simulink model "LICENTA_2024"  (R2018b)
settings: Solver=FixedStepDiscrete  StartTime=0.0  StopTime=Inf  RelTol=1e-3  EnableMultiTasking=on
values from neighbouring files (symbols this model uses):
  A = -Rs/Ld    (= -2.40983606557)    [licentam18.m]
  const_cuplu = 0.035    [licentam18.m]
  factor_conversie = (1/Rshunt)*(1/10)*(vref/4095)    (= 0.0115122972266)    [licentam18.m]
  FED = uint16(50)    [licentam18.m]
  MaxIter_1_ms_eCAP_wait = MinDetectSpeed_period/T_pos    (= 375)    [licentam18.m]
  pp = 16/2    (= 8)    [licentam18.m]
  RED = uint16(50)    [licentam18.m]
  T_pos = 0.0005    [licentam18.m]
  TBPRD1 = uint16(TPWM/(2*TTBCLK))    [licentam18.m]
  Tf = 0.015    [licentam18.m]
  Tf_spd = 0.01    [licentam18.m]
  Ts = Ts_crt_control    (= 3.33333333333e-05)    [licentam18.m]
  TTBCLK = 1/F    (= 5e-09)    [licentam18.m]
undefined symbols (not defined in the file or in its folder): Down, GPTRIP1SEL, GPTRIP2SEL, K, offset_ADC, radians, TZ1, TZ2, Up
libraries: tiiqmathlib x39, c2802xlib x9, c2837xDlib x6, simulink x5, c280xlib x4, c28xdmclib x2, c2000lib x1
(part 2 of 2)

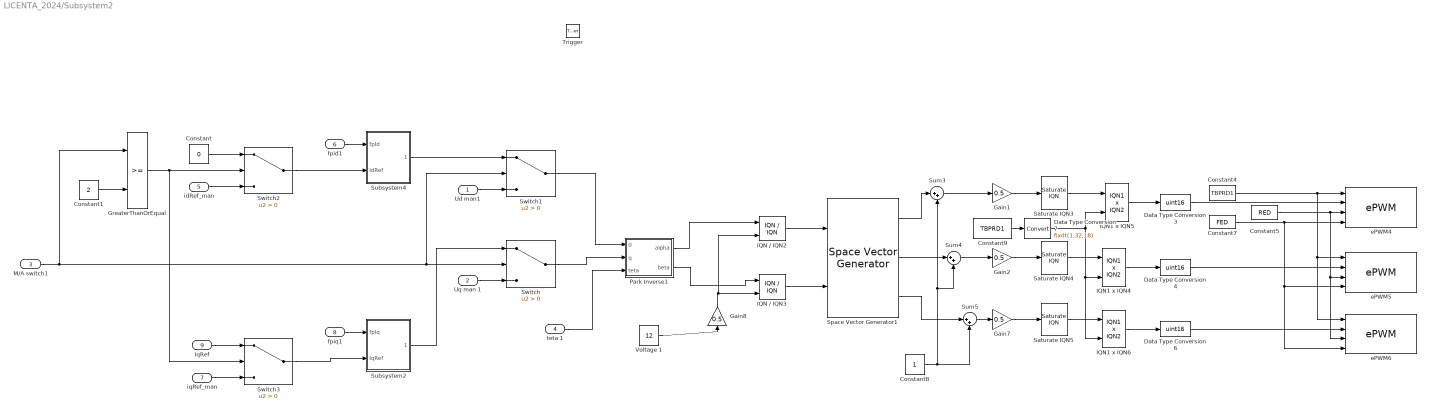
== system LICENTA_2024/Subsystem2 ==
  Ud man1 : Inport
  Uq man 1 : Inport  Port=2
  M/A switch1 : Inport  Port=3
  teta 1 : Inport  Port=4
  idRef_man : Inport  Port=5
  fpid1 : Inport  Port=6
  iqRef_man : Inport  Port=7
  fpiq1 : Inport  Port=8
  IqRef : Inport  Port=9
  Trigger : TriggerPort  TriggerType=function-call  VariantControl=Variant  PortDimensions=1
  Constant : Constant  Value=0
  Constant1 : Constant  Value=2
  Constant4 : Constant  Value=TBPRD1
  Constant5 : Constant  Value=RED
  Constant7 : Constant  Value=FED
  Constant8 : Constant  OutDataTypeStr=fixdt(1,32,24)
  Constant9 : Constant  Value=TBPRD1
  Data Type Conversion3 : DataTypeConversion  OutDataTypeStr=uint16
  Data Type Conversion4 : DataTypeConversion  OutDataTypeStr=uint16
  Data Type Conversion6 : DataTypeConversion  OutDataTypeStr=uint16
  Data Type Conversion7 : DataTypeConversion  OutDataTypeStr=fixdt(1,32,18)
  Gain{1..2,7..8} (4 alike) : Gain  Gain=0.5  OutDataTypeStr=Inherit: Same as input
  GreaterThanOrEqual : RelationalOperator  OutDataTypeStr=boolean  RndMeth=Simplest
  IQN / IQN2 : tiiqmathlib/IQN // IQN
      settings: SourceProductName=Embedded Coder Support Package for Texas Instruments C2000 Processors  SourceProductBaseCode=TIC2000
  IQN / IQN3 : tiiqmathlib/IQN // IQN
      settings: SourceProductName=Embedded Coder Support Package for Texas Instruments C2000 Processors  SourceProductBaseCode=TIC2000
  IQN1 x IQN4 : tiiqmathlib/IQN1 x IQN2  Q=10
      settings: SourceProductName=Embedded Coder Support Package for Texas Instruments C2000 Processors  SourceProductBaseCode=TIC2000
  IQN1 x IQN5 : tiiqmathlib/IQN1 x IQN2  Q=10
      settings: SourceProductName=Embedded Coder Support Package for Texas Instruments C2000 Processors  SourceProductBaseCode=TIC2000
  IQN1 x IQN6 : tiiqmathlib/IQN1 x IQN2  Q=10
      settings: SourceProductName=Embedded Coder Support Package for Texas Instruments C2000 Processors  SourceProductBaseCode=TIC2000
  Park Inverse1 : Subsystem
  Saturate IQN3 : tiiqmathlib/Saturate IQN  pos=0.95  neg=0.05
      settings: SourceProductName=Embedded Coder Support Package for Texas Instruments C2000 Processors  SourceProductBaseCode=TIC2000
  Saturate IQN4 : tiiqmathlib/Saturate IQN  pos=0.95  neg=0.05
      settings: SourceProductName=Embedded Coder Support Package for Texas Instruments C2000 Processors  SourceProductBaseCode=TIC2000
  Saturate IQN5 : tiiqmathlib/Saturate IQN  pos=0.95  neg=0.05
      settings: SourceProductName=Embedded Coder Support Package for Texas Instruments C2000 Processors  SourceProductBaseCode=TIC2000
  Space Vector Generator1 : c28xdmclib/Space Vector Generator
      settings: SourceProductName=Embedded Coder Support Package for Texas Instruments C2000 Processors  SourceProductBaseCode=TIC2000
  Subsystem2 : Subsystem
  Subsystem4 : Subsystem
  Sum3 : Sum  Inputs=|++
  Sum4 : Sum  Inputs=|++
  Sum5 : Sum  Inputs=|++
  Switch{,1..3} (4 alike) : Switch  Criteria=u2 > Threshold
  Voltage 1 : Constant  Value=12  OutDataTypeStr=fixdt(1,32,20)
  ePWM4 : c2802xlib/ePWM  useModule=ePWM1  ePWMxLINKTBPRD=Not Linked  periodUnits=Clock cycles  timerSource=Input port  timerPeriod_clk=TBPRD1+1  timerPeriod_sec=0.0001  tbshadow=Counter equals to zero  countingMode=Up-Down  phaseActiveEnable=Disable  phaseDirection=Count up after sync  phaseActive=0  synchronizationEnable=off  dcaevt1Sync=off  dcbevt1Sync=off  synchronizationOption=Counter equals to zero (CTR=Zero)  clockPrescale=1  HSclockPrescale=1  enswap=off  ePWMxAStatus=on  ePWMxAactionLogic1=Do nothing  ePWMxAactionLogic2=Do nothing  ePWMxAactionLogic3=Clear  ePWMxAactionLogic4=Set  ePWMxAactionLogic5=Do nothing  ePWMxAactionLogic6=Do nothing  ePWMxALoadMode=Load on counter equals to zero (CTR=Zero)  ePWMxACSFenable=off  ePWMxACSFvalue=Forcing disable  ePWMxASFreload=Zero  ePWMxBStatus=off  ePWMxBactionLogic1=Set  ePWMxBactionLogic2=Clear  ePWMxBactionLogic3=Do nothing  ePWMxBactionLogic4=Do nothing  ePWMxBactionLogic5=Clear  ePWMxBactionLogic6=Set  ePWMxBLoadMode=Load on counter equals to zero (CTR=Zero)  ePWMxBCSFenable=off  ePWMxBCSFvalue=Forcing disable  ePWMxBSFreload=Zero  ePWNxBOutWay=off  ePWMxLINKCMPA=Not Linked  CMPAUnits=Clock cycles  CMPASource=Input port  CMPAValue_per=50  CMPAValue_clk=0  enCMPAshadow=Counter equals to zero  ePWMxLINKCMPB=Not Linked  CMPBUnits=Clock cycles  CMPBSource=Specify via dialog  CMPBValue_per=50  CMPBValue_clk=0  enCMPBshadow=Counter equals to zero  ePWMxLINKCMPC=Not Linked  CMPCUnits=Clock cycles  CMPCSource=Specify via dialog  CMPCValue_per=50  CMPCValue_clk=32000  enCMPCshadow=Counter equals to zero  ePWMxLINKCMPD=Not Linked  CMPDUnits=Clock cycles  CMPDSource=Specify via dialog  CMPDValue_per=50  CMPDValue_clk=32000  enCMPDshadow=Counter equals to zero  enableDBePWMxA=on  enableDBePWMxB=on  enhalfcycle=off  DBpolarity=Active high complementary (AHC)  DBedgeDelay=Positive  DBSource_ePWMxA=ePWMxA  DBSource_ePWMxB=ePWMxA  DBperiodSource=Input port  REDperiod=0  FEDperiod=0  adcstartModuleA=on  adcrequestEventA=First event  adcstartEventA=Digital Compare Module A Event 1 start of conversion (DCAEVT1.soc)  adcstartEventA_type2=Counter equals to period (CTR=PRD)  adcstartModuleB=off  adcrequestEventB=First event  adcstartEventB=Counter equals to zero (CTR=Zero)  adcstartEventB_type2=Counter equals to zero (CTR=Zero)  intEn=off  intPrd=First event  intSel=Counter equals to zero (CTR=Zero)  intSel_type2=Counter equals to zero (CTR=Zero)  hrpe=off  enHRPWM=off  HRPWM_LoadMode=Counter equals to period (CTR=PRD)  HRPWM_CTLMode=Duty or Period control mode  HRPWM_EDGMode=Both edge  hrpeb=off  enHRPWMB=off  HRPWM_LoadModeB=Counter equals to zero (CTR=ZERO)  HRPWM_CTLModeB=Duty or Period control mode  HRPWM_EDGModeB=Both edge  enSFO=on  enautoconv=on  chopperEnable=off  chopperFrequency=1  chopperFirstwidth=1  chopperDuty=12.5%  tripZonesource=Specify via dialog  tzselOSHT1=off  tzselOSHT2=off  tzselOSHT3=off  tzselOSHDCAEV1=off  tzselOSHDCBEV1=off  tzselCBC1=off  tzselCBC2=off  tzselCBC3=off  tzselCBCDCAEV2=off  tzselCBCDCBEV2=off  tzselOSHT4=off  tzselOSHT5=off  tzselOSHT6=off  tzselCBC4=off  tzselCBC5=off  tzselCBC6=off  enTzOstIntr=off  enTzCbcIntr=off  enTzDCAEVT1Intr=off  enTzDCAEVT2Intr=off  enTzDCBEVT1Intr=off  enTzDCBEVT2Intr=off  ePWMxAforced=No action  ePWMxBforced=No action  DCAEVT1forced=No action  DCBEVT1forced=No action  DCAEVT2forced=No action  DCBEVT2forced=No action  dcah=Trip Zone 1 input (TZ1)  dcal=Trip Zone 2 input (TZ2)  dcbh=Trip Zone 1 input (TZ1)  dcbl=Trip Zone 2 input (TZ2)  dcah_type2=GPTRIP1SEL/(TZ1)  dcal_type2=GPTRIP2SEL/(TZ2)  dcbh_type2=GPTRIP1SEL/(TZ1)  dcbl_type2=GPTRIP2SEL/(TZ2)  gendcaevt1=Event disabled  gendcaevt2=Event disabled  gendcbevt1=Event disabled  gendcbevt2=Event disabled  dcaevt1src=DCAEVT1 with sync  dcaevt2src=DCAEVT2 with sync  dcbevt1src=DCBEVT1 with sync  dcbevt2src=DCBEVT2 with sync  pulsesel=Counter equals to zero (CTR=Zero)  blankinv=off  blankoffset=0  blankwidth=0  evsrcsel=Filtered version of DCAEVT1 (DCAEVT1FILT)  encape=off  PwmType=C2000_Type4
      settings: SourceProductName=Embedded Coder Support Package for Texas Instruments C2000 Processors
  ePWM5 : c2802xlib/ePWM  useModule=ePWM2  ePWMxLINKTBPRD=Not Linked  periodUnits=Clock cycles  timerSource=Input port  timerPeriod_clk=TBPRD1+1  timerPeriod_sec=0.0001  tbshadow=Counter equals to zero  countingMode=Up-Down  phaseActiveEnable=Disable  phaseDirection=Count up after sync  phaseActive=0  synchronizationEnable=off  dcaevt1Sync=off  dcbevt1Sync=off  synchronizationOption=Counter equals to zero (CTR=Zero)  clockPrescale=1  HSclockPrescale=1  enswap=off  ePWMxAStatus=on  ePWMxAactionLogic1=Do nothing  ePWMxAactionLogic2=Do nothing  ePWMxAactionLogic3=Clear  ePWMxAactionLogic4=Set  ePWMxAactionLogic5=Do nothing  ePWMxAactionLogic6=Do nothing  ePWMxALoadMode=Load on counter equals to zero (CTR=Zero)  ePWMxACSFenable=off  ePWMxACSFvalue=Forcing disable  ePWMxASFreload=Zero  ePWMxBStatus=off  ePWMxBactionLogic1=Set  ePWMxBactionLogic2=Clear  ePWMxBactionLogic3=Do nothing  ePWMxBactionLogic4=Do nothing  ePWMxBactionLogic5=Clear  ePWMxBactionLogic6=Set  ePWMxBLoadMode=Load on counter equals to zero (CTR=Zero)  ePWMxBCSFenable=off  ePWMxBCSFvalue=Forcing disable  ePWMxBSFreload=Zero  ePWNxBOutWay=off  ePWMxLINKCMPA=Not Linked  CMPAUnits=Clock cycles  CMPASource=Input port  CMPAValue_per=50  CMPAValue_clk=0  enCMPAshadow=Counter equals to zero  ePWMxLINKCMPB=Not Linked  CMPBUnits=Clock cycles  CMPBSource=Specify via dialog  CMPBValue_per=50  CMPBValue_clk=0  enCMPBshadow=Counter equals to zero  ePWMxLINKCMPC=Not Linked  CMPCUnits=Clock cycles  CMPCSource=Specify via dialog  CMPCValue_per=50  CMPCValue_clk=32000  enCMPCshadow=Counter equals to zero  ePWMxLINKCMPD=Not Linked  CMPDUnits=Clock cycles  CMPDSource=Specify via dialog  CMPDValue_per=50  CMPDValue_clk=32000  enCMPDshadow=Counter equals to zero  enableDBePWMxA=on  enableDBePWMxB=on  enhalfcycle=off  DBpolarity=Active high complementary (AHC)  DBedgeDelay=Positive  DBSource_ePWMxA=ePWMxA  DBSource_ePWMxB=ePWMxA  DBperiodSource=Input port  REDperiod=0  FEDperiod=0  adcstartModuleA=on  adcrequestEventA=First event  adcstartEventA=Digital Compare Module A Event 1 start of conversion (DCAEVT1.soc)  adcstartEventA_type2=Counter equals to period (CTR=PRD)  adcstartModuleB=off  adcrequestEventB=First event  adcstartEventB=Counter equals to zero (CTR=Zero)  adcstartEventB_type2=Counter equals to zero (CTR=Zero)  intEn=off  intPrd=First event  intSel=Counter equals to zero (CTR=Zero)  intSel_type2=Counter equals to zero (CTR=Zero)  hrpe=off  enHRPWM=off  HRPWM_LoadMode=Counter equals to period (CTR=PRD)  HRPWM_CTLMode=Duty or Period control mode  HRPWM_EDGMode=Both edge  hrpeb=off  enHRPWMB=off  HRPWM_LoadModeB=Counter equals to zero (CTR=ZERO)  HRPWM_CTLModeB=Duty or Period control mode  HRPWM_EDGModeB=Both edge  enSFO=on  enautoconv=on  chopperEnable=off  chopperFrequency=1  chopperFirstwidth=1  chopperDuty=12.5%  tripZonesource=Specify via dialog  tzselOSHT1=off  tzselOSHT2=off  tzselOSHT3=off  tzselOSHDCAEV1=off  tzselOSHDCBEV1=off  tzselCBC1=off  tzselCBC2=off  tzselCBC3=off  tzselCBCDCAEV2=off  tzselCBCDCBEV2=off  tzselOSHT4=off  tzselOSHT5=off  tzselOSHT6=off  tzselCBC4=off  tzselCBC5=off  tzselCBC6=off  enTzOstIntr=off  enTzCbcIntr=off  enTzDCAEVT1Intr=off  enTzDCAEVT2Intr=off  enTzDCBEVT1Intr=off  enTzDCBEVT2Intr=off  ePWMxAforced=No action  ePWMxBforced=No action  DCAEVT1forced=No action  DCBEVT1forced=No action  DCAEVT2forced=No action  DCBEVT2forced=No action  dcah=Trip Zone 1 input (TZ1)  dcal=Trip Zone 2 input (TZ2)  dcbh=Trip Zone 1 input (TZ1)  dcbl=Trip Zone 2 input (TZ2)  dcah_type2=GPTRIP1SEL/(TZ1)  dcal_type2=GPTRIP2SEL/(TZ2)  dcbh_type2=GPTRIP1SEL/(TZ1)  dcbl_type2=GPTRIP2SEL/(TZ2)  gendcaevt1=Event disabled  gendcaevt2=Event disabled  gendcbevt1=Event disabled  gendcbevt2=Event disabled  dcaevt1src=DCAEVT1 with sync  dcaevt2src=DCAEVT2 with sync  dcbevt1src=DCBEVT1 with sync  dcbevt2src=DCBEVT2 with sync  pulsesel=Counter equals to zero (CTR=Zero)  blankinv=off  blankoffset=0  blankwidth=0  evsrcsel=Filtered version of DCAEVT1 (DCAEVT1FILT)  encape=off  PwmType=C2000_Type4
      settings: SourceProductName=Embedded Coder Support Package for Texas Instruments C2000 Processors
  ePWM6 : c2802xlib/ePWM  useModule=ePWM3  ePWMxLINKTBPRD=Not Linked  periodUnits=Clock cycles  timerSource=Input port  timerPeriod_clk=TBPRD1+1  timerPeriod_sec=0.0001  tbshadow=Counter equals to zero  countingMode=Up-Down  phaseActiveEnable=Disable  phaseDirection=Count up after sync  phaseActive=0  synchronizationEnable=off  dcaevt1Sync=off  dcbevt1Sync=off  synchronizationOption=Counter equals to zero (CTR=Zero)  clockPrescale=1  HSclockPrescale=1  enswap=off  ePWMxAStatus=on  ePWMxAactionLogic1=Do nothing  ePWMxAactionLogic2=Do nothing  ePWMxAactionLogic3=Clear  ePWMxAactionLogic4=Set  ePWMxAactionLogic5=Do nothing  ePWMxAactionLogic6=Do nothing  ePWMxALoadMode=Load on counter equals to zero (CTR=Zero)  ePWMxACSFenable=off  ePWMxACSFvalue=Forcing disable  ePWMxASFreload=Zero  ePWMxBStatus=off  ePWMxBactionLogic1=Set  ePWMxBactionLogic2=Clear  ePWMxBactionLogic3=Do nothing  ePWMxBactionLogic4=Do nothing  ePWMxBactionLogic5=Clear  ePWMxBactionLogic6=Set  ePWMxBLoadMode=Load on counter equals to zero (CTR=Zero)  ePWMxBCSFenable=off  ePWMxBCSFvalue=Forcing disable  ePWMxBSFreload=Zero  ePWNxBOutWay=off  ePWMxLINKCMPA=Not Linked  CMPAUnits=Clock cycles  CMPASource=Input port  CMPAValue_per=50  CMPAValue_clk=0  enCMPAshadow=Counter equals to zero  ePWMxLINKCMPB=Not Linked  CMPBUnits=Clock cycles  CMPBSource=Specify via dialog  CMPBValue_per=50  CMPBValue_clk=0  enCMPBshadow=Counter equals to zero  ePWMxLINKCMPC=Not Linked  CMPCUnits=Clock cycles  CMPCSource=Specify via dialog  CMPCValue_per=50  CMPCValue_clk=32000  enCMPCshadow=Counter equals to zero  ePWMxLINKCMPD=Not Linked  CMPDUnits=Clock cycles  CMPDSource=Specify via dialog  CMPDValue_per=50  CMPDValue_clk=32000  enCMPDshadow=Counter equals to zero  enableDBePWMxA=on  enableDBePWMxB=on  enhalfcycle=off  DBpolarity=Active high complementary (AHC)  DBedgeDelay=Positive  DBSource_ePWMxA=ePWMxA  DBSource_ePWMxB=ePWMxA  DBperiodSource=Input port  REDperiod=0  FEDperiod=0  adcstartModuleA=on  adcrequestEventA=First event  adcstartEventA=Digital Compare Module A Event 1 start of conversion (DCAEVT1.soc)  adcstartEventA_type2=Counter equals to period (CTR=PRD)  adcstartModuleB=off  adcrequestEventB=First event  adcstartEventB=Counter equals to zero (CTR=Zero)  adcstartEventB_type2=Counter equals to zero (CTR=Zero)  intEn=off  intPrd=First event  intSel=Counter equals to zero (CTR=Zero)  intSel_type2=Counter equals to zero (CTR=Zero)  hrpe=off  enHRPWM=off  HRPWM_LoadMode=Counter equals to period (CTR=PRD)  HRPWM_CTLMode=Duty or Period control mode  HRPWM_EDGMode=Both edge  hrpeb=off  enHRPWMB=off  HRPWM_LoadModeB=Counter equals to zero (CTR=ZERO)  HRPWM_CTLModeB=Duty or Period control mode  HRPWM_EDGModeB=Both edge  enSFO=on  enautoconv=on  chopperEnable=off  chopperFrequency=1  chopperFirstwidth=1  chopperDuty=12.5%  tripZonesource=Specify via dialog  tzselOSHT1=off  tzselOSHT2=off  tzselOSHT3=off  tzselOSHDCAEV1=off  tzselOSHDCBEV1=off  tzselCBC1=off  tzselCBC2=off  tzselCBC3=off  tzselCBCDCAEV2=off  tzselCBCDCBEV2=off  tzselOSHT4=off  tzselOSHT5=off  tzselOSHT6=off  tzselCBC4=off  tzselCBC5=off  tzselCBC6=off  enTzOstIntr=off  enTzCbcIntr=off  enTzDCAEVT1Intr=off  enTzDCAEVT2Intr=off  enTzDCBEVT1Intr=off  enTzDCBEVT2Intr=off  ePWMxAforced=No action  ePWMxBforced=No action  DCAEVT1forced=No action  DCBEVT1forced=No action  DCAEVT2forced=No action  DCBEVT2forced=No action  dcah=Trip Zone 1 input (TZ1)  dcal=Trip Zone 2 input (TZ2)  dcbh=Trip Zone 1 input (TZ1)  dcbl=Trip Zone 2 input (TZ2)  dcah_type2=GPTRIP1SEL/(TZ1)  dcal_type2=GPTRIP2SEL/(TZ2)  dcbh_type2=GPTRIP1SEL/(TZ1)  dcbl_type2=GPTRIP2SEL/(TZ2)  gendcaevt1=Event disabled  gendcaevt2=Event disabled  gendcbevt1=Event disabled  gendcbevt2=Event disabled  dcaevt1src=DCAEVT1 with sync  dcaevt2src=DCAEVT2 with sync  dcbevt1src=DCBEVT1 with sync  dcbevt2src=DCBEVT2 with sync  pulsesel=Counter equals to zero (CTR=Zero)  blankinv=off  blankoffset=0  blankwidth=0  evsrcsel=Filtered version of DCAEVT1 (DCAEVT1FILT)  encape=off  PwmType=C2000_Type4
      settings: SourceProductName=Embedded Coder Support Package for Texas Instruments C2000 Processors
  wires:
  Sum4/1 -> Gain2/1
  Data Type Conversion3/1 -> ePWM4/2
  Voltage 1/1 -> Gain8/1
  IQN1 x IQN5/1 -> Data Type Conversion3/1
  Space Vector Generator1/3 -> Sum5/1
  Constant5/1 -> ePWM6/3, ePWM5/3, ePWM4/3
  Saturate IQN4/1 -> IQN1 x IQN4/1
  Saturate IQN3/1 -> IQN1 x IQN5/1
  Gain8/1 -> IQN / IQN3/2, IQN / IQN2/2
  Data Type Conversion6/1 -> ePWM6/2
  Sum3/1 -> Gain1/1
  Gain1/1 -> Saturate IQN3/1
  Space Vector Generator1/1 -> Sum3/1
  Space Vector Generator1/2 -> Sum4/1
  Data Type Conversion7/1 -> IQN1 x IQN5/2, IQN1 x IQN6/2, IQN1 x IQN4/2
  Constant7/1 -> ePWM6/4, ePWM5/4, ePWM4/4
  IQN1 x IQN4/1 -> Data Type Conversion4/1
  Saturate IQN5/1 -> IQN1 x IQN6/1
  teta 1/1 -> Park Inverse1/3(teta)
  Park Inverse1/2(beta) -> IQN / IQN3/1
  Data Type Conversion4/1 -> ePWM5/2
  IQN1 x IQN6/1 -> Data Type Conversion6/1
  Park Inverse1/1(alpha) -> IQN / IQN2/1
  Gain2/1 -> Saturate IQN4/1
  Constant8/1 -> Sum4/2, Sum3/2, Sum5/2
  IQN / IQN2/1 -> Space Vector Generator1/1
  Sum5/1 -> Gain7/1
  IQN / IQN3/1 -> Space Vector Generator1/2
  fpid1/1 -> Subsystem4/1(fpId)
  fpiq1/1 -> Subsystem2/1(fpIq)
  Gain7/1 -> Saturate IQN5/1
  Constant9/1 -> Data Type Conversion7/1
  Constant4/1 -> ePWM6/1, ePWM5/1, ePWM4/1
  Switch1/1 -> Park Inverse1/1(d)
  Ud man1/1 -> Switch1/3
  Uq man 1/1 -> Switch/3
  Switch/1 -> Park Inverse1/2(q)
  Subsystem2/1(Uq LQR1) -> Switch/1
  Subsystem4/1(Ud LQR1) -> Switch1/1
  Switch2/1 -> Subsystem4/2(IdRef)
  Switch3/1 -> Subsystem2/2(IqRef)
  Constant/1 -> Switch2/1
  idRef_man/1 -> Switch2/3
  iqRef_man/1 -> Switch3/3
  Constant1/1 -> GreaterThanOrEqual/2
  GreaterThanOrEqual/1 -> Switch3/2, Switch2/2
  M/A switch1/1 -> GreaterThanOrEqual/1, Switch1/2, Switch/2
  IqRef/1 -> Switch3/1

== system LICENTA_2024/Subsystem3 ==
  fpiq : Inport
  iqRef : Inport  Port=2
  Ki : Inport  Port=3
  Kp : Inport  Port=4
  Trigger : TriggerPort  TriggerType=function-call  VariantControl=Variant  PortDimensions=1
  Subsystem5 : Subsystem
  regulator curent iq : Subsystem
  IqRef : Outport
  wires:
  regulator curent iq/1(Uq PI1) -> Subsystem5/1("torque_Ref ")
  fpiq/1 -> regulator curent iq/4(fpiq)
  iqRef/1 -> regulator curent iq/3(iqRef)
  Ki/1 -> regulator curent iq/1(KiPI)
  Kp/1 -> regulator curent iq/2(KpPI)
  Subsystem5/1(IqRef) -> IqRef/1

== system LICENTA_2024/calc pozitiei si a vitezei ==
  bToggleInterruptECAP : Inport
  FrqHzElec : Inport  Port=2
  In3 : Inport  Port=3
  Trigger : TriggerPort  TriggerType=function-call  VariantControl=(inherit)  PortDimensions=1
  Terminator{,1..3,5} (5 alike) : Terminator
  calc pozitie : Subsystem
  calc viteza : Subsystem
  teta : Outport  VectorParamsAs1DForOutWhenUnconnected=on
  RPMSpdFil : Outport  Port=2  VectorParamsAs1DForOutWhenUnconnected=on
  wires:
  bToggleInterruptECAP/1 -> calc viteza/3(bToggleInterruptECAP)
  calc viteza/1(RPMSpdFil) -> RPMSpdFil/1
  FrqHzElec/1 -> calc viteza/2(FrqHzElec)
  calc pozitie/2(int8dir) -> calc viteza/1(int8Dir)
  calc viteza/2(HzHallFreqFil) -> Terminator/1
  calc viteza/3(RadpsMechFreqFil) -> Terminator1/1
  calc viteza/4(RadpsHallFreq) -> Terminator2/1
  calc viteza/5(RadpsHallFreqFil) -> Terminator3/1
  calc viteza/6(bSPDNOTDetected) -> Terminator5/1
  calc pozitie/1(teta) -> teta/1
  In3/1 -> calc pozitie/1(In1)

== system LICENTA_2024/eCAP ==
  Post interrupt on capture event 1() : TriggerPort  TriggerType=function-call  VariantControl=(inherit)  PortDimensions=1
  Data Type Conversion : DataTypeConversion  OutDataTypeStr=uint32
  Data Type Conversion1 : DataTypeConversion  OutDataTypeStr=uint32
  Gain : Gain  Gain=TTBCLK
  If : If  IfExpression=u1 <= Min_eCAP  ElseIfExpressions=u1 >= Max_eCAP
  If Action Subsystem : Subsystem  TreatAsAtomicUnit=on
  If Action Subsystem1 : Subsystem  TreatAsAtomicUnit=on
  If Action Subsystem2 : Subsystem  TreatAsAtomicUnit=on
  Max : MinMax  Function=max  Inputs=2
  Merge : Merge  Inputs=3
  NOT : Logic  Operator=NOT  IconShape=distinctive  AllPortsSameDT=off  OutDataTypeStr=boolean
  Unit Delay : UnitDelay  SampleTime=-1
  Unit Delay1 : UnitDelay  SampleTime=-1
  "eCAP1 " : c280xlib/eCAP  operatingMode=eCAP  selectCAPx=eCAP1  offsetValue=0  counterSynIn=off  enableCounter=off  syncOutput=Disabled  sampleTime=-1  eventPrescaler=0  selectMode=Continuous  enableOneShot=off  stopValue=Capture Event 1  resetEv1Ts=on  ev1Polarity=Rising Edge  resetEv2Ts=off  ev2Polarity=Rising Edge  resetEv3Ts=off  ev3Polarity=Rising Edge  resetEv4Ts=off  ev4Polarity=Rising Edge  tSCntrDataType=single  capEvFlag=off  capFlagDataType=uint16  overFlowFlag=off  overFlowFlagDataType=uint16  periodUnit=Seconds  periodSource=Specify via dialog  waveformPeriod=0.001  dutyUnit=Percentages  dutySource=Specify via dialog  dutyCycle=50  outputPolarity=Active High  enableCEVT1Int=on  enableCEVT2Int=off  enableCEVT3Int=off  enableCEVT4Int=off  enableCTROVFInt=off  enablePRDInt=off  enableCMPInt=off
      settings: SourceProductBaseCode=TIC2000
  "eCAP2 " : c280xlib/eCAP  operatingMode=eCAP  selectCAPx=eCAP2  offsetValue=0  counterSynIn=off  enableCounter=off  syncOutput=Disabled  sampleTime=-1  eventPrescaler=0  selectMode=Continuous  enableOneShot=off  stopValue=Capture Event 1  resetEv1Ts=on  ev1Polarity=Rising Edge  resetEv2Ts=off  ev2Polarity=Rising Edge  resetEv3Ts=off  ev3Polarity=Rising Edge  resetEv4Ts=off  ev4Polarity=Rising Edge  tSCntrDataType=single  capEvFlag=off  capFlagDataType=uint16  overFlowFlag=off  overFlowFlagDataType=uint16  periodUnit=Seconds  periodSource=Specify via dialog  waveformPeriod=0.001  dutyUnit=Percentages  dutySource=Specify via dialog  dutyCycle=50  outputPolarity=Active High  enableCEVT1Int=on  enableCEVT2Int=off  enableCEVT3Int=off  enableCEVT4Int=off  enableCTROVFInt=off  enablePRDInt=off  enableCMPInt=off
      settings: SourceProductBaseCode=TIC2000
  FrqHzElec : Outport
  bToggleInterruptECAP : Outport  Port=2
  wires:
  NOT/1 -> bToggleInterruptECAP/1, Unit Delay1/1
  Unit Delay1/1 -> NOT/1
  Unit Delay/1 -> If Action Subsystem/1(HzHallFreqPrev)
  Merge/1 -> FrqHzElec/1, Unit Delay/1
  Gain/1 -> If Action Subsystem2/1(HallPeriod)
  If Action Subsystem2/1(HzHallFreq) -> Merge/3
  If Action Subsystem1/1(HzHallFreq) -> Merge/2
  If Action Subsystem/1(HzHallFreq) -> Merge/1
  If/3 -> If Action Subsystem2/Action
  If/2 -> If Action Subsystem1/Action
  If/1 -> If Action Subsystem/Action
  Max/1 -> If/1, Gain/1
  Data Type Conversion1/1 -> Max/1
  Data Type Conversion/1 -> Max/2
  "eCAP1 "/1 -> Data Type Conversion1/1
  "eCAP2 "/1 -> Data Type Conversion/1

== system LICENTA_2024/PWM/Park Inverse ==
  d : Inport
  q : Inport  Port=2
  teta : Inport  Port=3
  Data Type Conversion : DataTypeConversion  OutDataTypeStr=fixdt(1,32,20)
  Data Type Conversion1 : DataTypeConversion  OutDataTypeStr=fixdt(1,32,20)
  IQN1 x IQN{1..4} (4 alike) : tiiqmathlib/IQN1 x IQN2  Q=20
      settings: SourceProductName=Embedded Coder Support Package for Texas Instruments C2000 Processors  SourceProductBaseCode=TIC2000
  Sum1 : Sum  Inputs=|++  OutDataTypeStr=Inherit: Same as first input
  Sum2 : Sum  Inputs=|+-  OutDataTypeStr=Inherit: Same as first input
  cos IQN : tiiqmathlib/Trig Fcn IQN  functionOption=_IQcos
      settings: SourceProductName=Embedded Coder Support Package for Texas Instruments C2000 Processors  SourceProductBaseCode=TIC2000
  sin IQN : tiiqmathlib/Trig Fcn IQN  functionOption=_IQsin
      settings: SourceProductName=Embedded Coder Support Package for Texas Instruments C2000 Processors  SourceProductBaseCode=TIC2000
  alpha : Outport
  beta : Outport  Port=2
  wires:
  teta/1 -> cos IQN/1, sin IQN/1
  Sum2/1 -> alpha/1
  d/1 -> Data Type Conversion/1
  sin IQN/1 -> IQN1 x IQN4/2, IQN1 x IQN1/2
  cos IQN/1 -> IQN1 x IQN3/2, IQN1 x IQN2/2
  q/1 -> Data Type Conversion1/1
  Sum1/1 -> beta/1
  IQN1 x IQN2/1 -> Sum2/1
  IQN1 x IQN1/1 -> Sum2/2
  IQN1 x IQN3/1 -> Sum1/1
  IQN1 x IQN4/1 -> Sum1/2
  Data Type Conversion/1 -> IQN1 x IQN4/1, IQN1 x IQN2/1
  Data Type Conversion1/1 -> IQN1 x IQN3/1, IQN1 x IQN1/1

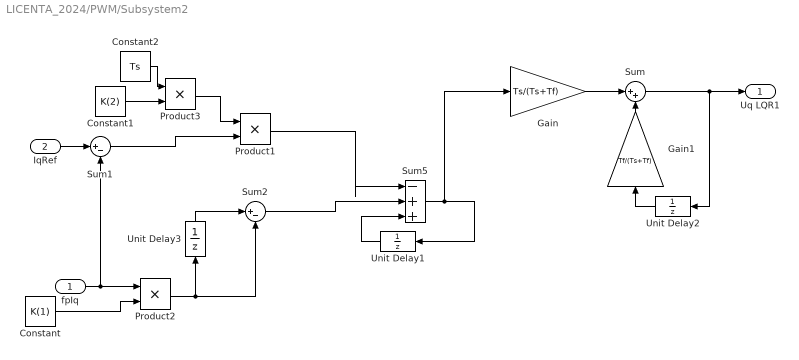
== system LICENTA_2024/PWM/Subsystem2 ==
  fpIq : Inport
  IqRef : Inport  Port=2
  Constant : Constant  Value=K(1)
  Constant1 : Constant  Value=K(2)
  Constant2 : Constant  Value=Ts
  Gain : Gain  Gain=Ts/(Ts+Tf)
  Gain1 : Gain  Gain=Tf/(Ts+Tf)
  Product1 : Product
  Product2 : Product
  Product3 : Product
  Sum : Sum  Inputs=|++
  Sum1 : Sum  Inputs=|+-
  Sum2 : Sum  Inputs=|+-
  Sum5 : Sum  Inputs=|-++
  Unit Delay1 : UnitDelay  SampleTime=-1
  Unit Delay2 : UnitDelay  SampleTime=-1
  Unit Delay3 : UnitDelay  SampleTime=-1
  Uq LQR1 : Outport
  wires:
  Product1/1 -> Sum5/1
  fpIq/1 -> Product2/1, Sum1/2
  Product3/1 -> Product1/1
  Constant/1 -> Product2/2
  Constant2/1 -> Product3/1
  Unit Delay3/1 -> Sum2/1
  Product2/1 -> Unit Delay3/1, Sum2/2
  Unit Delay1/1 -> Sum5/3
  Constant1/1 -> Product3/2
  IqRef/1 -> Sum1/1
  Sum1/1 -> Product1/2
  Sum2/1 -> Sum5/2
  Gain1/1 -> Sum/2
  Gain/1 -> Sum/1
  Unit Delay2/1 -> Gain1/1
  Sum/1 -> Uq LQR1/1, Unit Delay2/1
  Sum5/1 -> Unit Delay1/1, Gain/1

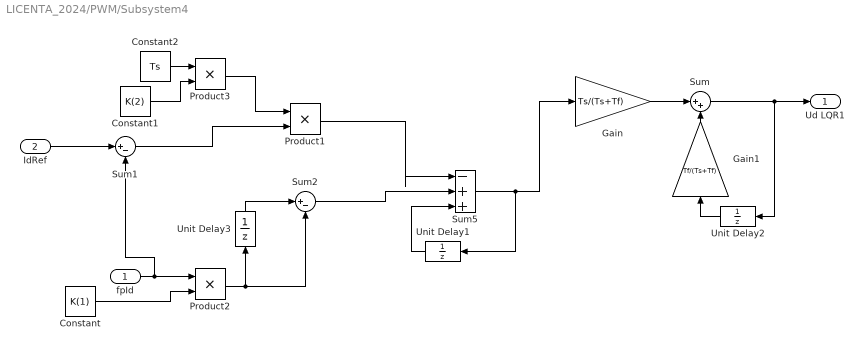
== system LICENTA_2024/PWM/Subsystem4 ==
  fpId : Inport
  IdRef : Inport  Port=2
  Constant : Constant  Value=K(1)
  Constant1 : Constant  Value=K(2)
  Constant2 : Constant  Value=Ts
  Gain : Gain  Gain=Ts/(Ts+Tf)
  Gain1 : Gain  Gain=Tf/(Ts+Tf)
  Product1 : Product
  Product2 : Product
  Product3 : Product
  Sum : Sum  Inputs=|++
  Sum1 : Sum  Inputs=|+-
  Sum2 : Sum  Inputs=|+-
  Sum5 : Sum  Inputs=|-++
  Unit Delay1 : UnitDelay  SampleTime=-1
  Unit Delay2 : UnitDelay  SampleTime=-1
  Unit Delay3 : UnitDelay  SampleTime=-1
  Ud LQR1 : Outport
  wires:
  Sum5/1 -> Unit Delay1/1, Gain/1
  Unit Delay1/1 -> Sum5/3
  Product2/1 -> Sum2/2, Unit Delay3/1
  Unit Delay3/1 -> Sum2/1
  Constant2/1 -> Product3/1
  Constant/1 -> Product2/2
  Product3/1 -> Product1/1
  fpId/1 -> Product2/1, Sum1/2
  Product1/1 -> Sum5/1
  Constant1/1 -> Product3/2
  IdRef/1 -> Sum1/1
  Sum1/1 -> Product1/2
  Sum2/1 -> Sum5/2
  Unit Delay2/1 -> Gain1/1
  Gain1/1 -> Sum/2
  Gain/1 -> Sum/1
  Sum/1 -> Ud LQR1/1, Unit Delay2/1

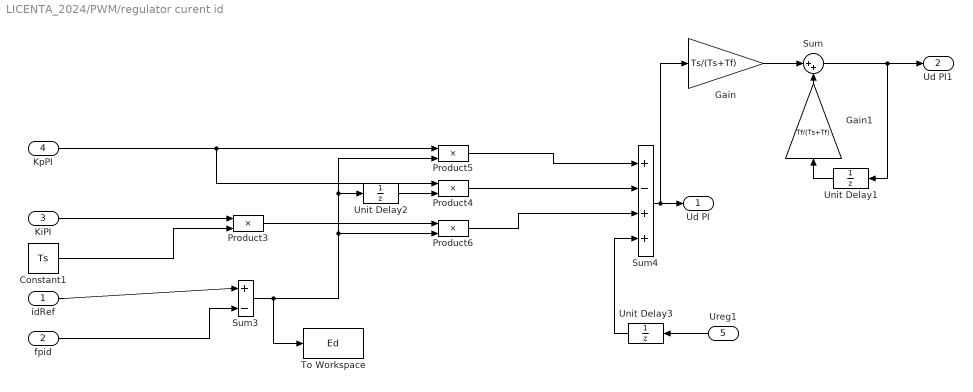
== system LICENTA_2024/PWM/regulator curent id ==
  idRef : Inport
  fpid : Inport  Port=2
  KiPI : Inport  Port=3
  KpPI : Inport  Port=4
  Ureg1 : Inport  Port=5
  Constant1 : Constant  Value=Ts  OutDataTypeStr=single  SampleTime=-1
  Gain : Gain  Gain=Ts/(Ts+Tf)
  Gain1 : Gain  Gain=Tf/(Ts+Tf)
  Product{3..6} (4 alike) : Product
  Sum : Sum  Inputs=|++
  Sum3 : Sum  Inputs=|+-
  Sum4 : Sum  Inputs=+-++
  To Workspace : ToWorkspace  VariableName=Ed  SaveFormat=Timeseries  SampleTime=-1
  Unit Delay1 : UnitDelay  SampleTime=-1
  Unit Delay2 : UnitDelay  SampleTime=-1
  Unit Delay3 : UnitDelay  SampleTime=-1
  Ud PI : Outport
  Ud PI1 : Outport  Port=2
  wires:
  Product5/1 -> Sum4/1
  Product6/1 -> Sum4/3
  KpPI/1 -> Product4/1, Product5/1
  Ureg1/1 -> Unit Delay3/1
  Product4/1 -> Sum4/2
  Unit Delay3/1 -> Sum4/4
  Constant1/1 -> Product3/2
  idRef/1 -> Sum3/1
  KiPI/1 -> Product3/1
  fpid/1 -> Sum3/2
  Sum3/1 -> To Workspace/1, Product6/2, Product5/2, Unit Delay2/1
  Product3/1 -> Product6/1
  Gain1/1 -> Sum/2
  Gain/1 -> Sum/1
  Unit Delay1/1 -> Gain1/1
  Sum/1 -> Ud PI1/1, Unit Delay1/1
  Sum4/1 -> Gain/1, Ud PI/1
  Unit Delay2/1 -> Product4/2

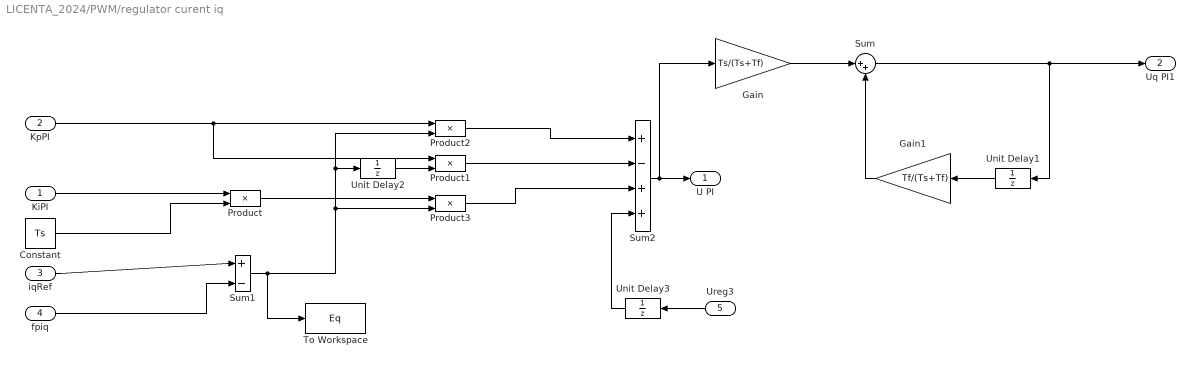
== system LICENTA_2024/PWM/regulator curent iq ==
  KiPI : Inport
  KpPI : Inport  Port=2
  iqRef : Inport  Port=3
  fpiq : Inport  Port=4
  Ureg3 : Inport  Port=5
  Constant : Constant  Value=Ts  OutDataTypeStr=single  SampleTime=-1
  Gain : Gain  Gain=Ts/(Ts+Tf)
  Gain1 : Gain  Gain=Tf/(Ts+Tf)
  Product{,1..3} (4 alike) : Product
  Sum : Sum  Inputs=|++
  Sum1 : Sum  Inputs=|+-
  Sum2 : Sum  Inputs=+-++
  To Workspace : ToWorkspace  VariableName=Eq  SaveFormat=Timeseries  SampleTime=-1
  Unit Delay1 : UnitDelay  SampleTime=-1
  Unit Delay2 : UnitDelay  SampleTime=-1
  Unit Delay3 : UnitDelay  SampleTime=-1
  U PI : Outport
  Uq PI1 : Outport  Port=2
  wires:
  Sum2/1 -> Gain/1, U PI/1
  Sum1/1 -> To Workspace/1, Product3/2, Product2/2, Unit Delay2/1
  fpiq/1 -> Sum1/2
  iqRef/1 -> Sum1/1
  KiPI/1 -> Product/1
  Constant/1 -> Product/2
  Ureg3/1 -> Unit Delay3/1
  Unit Delay3/1 -> Sum2/4
  Product2/1 -> Sum2/1
  KpPI/1 -> Product1/1, Product2/1
  Product1/1 -> Sum2/2
  Product3/1 -> Sum2/3
  Product/1 -> Product3/1
  Gain/1 -> Sum/1
  Sum/1 -> Uq PI1/1, Unit Delay1/1
  Unit Delay1/1 -> Gain1/1
  Gain1/1 -> Sum/2
  Unit Delay2/1 -> Product1/2

== system LICENTA_2024/Subsystem/3value average ==
  in : Inport
  Gain : Gain  Gain=1/3  OutDataTypeStr=fixdt(1,32,16)
  Sum : Sum  Inputs=3
  Unit Delay : UnitDelay  SampleTime=-1
  Unit Delay1 : UnitDelay  SampleTime=-1
  out : Outport
  wires:
  Sum/1 -> Gain/1
  Gain/1 -> out/1
  in/1 -> Unit Delay1/1, Sum/1
  Unit Delay1/1 -> Sum/2, Unit Delay/1
  Unit Delay/1 -> Sum/3

== system LICENTA_2024/Subsystem/3value average1 ==
  in : Inport
  Gain : Gain  Gain=1/3  OutDataTypeStr=fixdt(1,32,16)
  Sum : Sum  Inputs=3
  Unit Delay : UnitDelay  SampleTime=-1
  Unit Delay1 : UnitDelay  SampleTime=-1
  out : Outport
  wires:
  Unit Delay/1 -> Sum/3
  Unit Delay1/1 -> Unit Delay/1, Sum/2
  in/1 -> Sum/1, Unit Delay1/1
  Gain/1 -> out/1
  Sum/1 -> Gain/1

== system LICENTA_2024/Subsystem/3value average2 ==
  in : Inport
  Gain : Gain  Gain=1/3  OutDataTypeStr=fixdt(1,32,16)
  Sum : Sum  Inputs=3
  Unit Delay : UnitDelay  SampleTime=-1
  Unit Delay1 : UnitDelay  SampleTime=-1
  out : Outport
  wires:
  Unit Delay/1 -> Sum/3
  Unit Delay1/1 -> Unit Delay/1, Sum/2
  in/1 -> Sum/1, Unit Delay1/1
  Gain/1 -> out/1
  Sum/1 -> Gain/1

== system LICENTA_2024/Subsystem/3value average3 ==
  in : Inport
  Gain : Gain  Gain=1/3  OutDataTypeStr=fixdt(1,32,16)
  Sum : Sum  Inputs=3
  Unit Delay : UnitDelay  SampleTime=-1
  Unit Delay1 : UnitDelay  SampleTime=-1
  out : Outport
  wires:
  Sum/1 -> Gain/1
  Gain/1 -> out/1
  in/1 -> Unit Delay1/1, Sum/1
  Unit Delay1/1 -> Sum/2, Unit Delay/1
  Unit Delay/1 -> Sum/3

== system LICENTA_2024/Subsystem/3value average4 ==
  in : Inport
  Gain : Gain  Gain=1/3  OutDataTypeStr=fixdt(1,32,16)
  Sum : Sum  Inputs=3
  Unit Delay : UnitDelay  SampleTime=-1
  Unit Delay1 : UnitDelay  SampleTime=-1
  out : Outport
  wires:
  Sum/1 -> Gain/1
  Gain/1 -> out/1
  in/1 -> Unit Delay1/1, Sum/1
  Unit Delay1/1 -> Sum/2, Unit Delay/1
  Unit Delay/1 -> Sum/3

== system LICENTA_2024/Subsystem/transf clarke ==
  fISENA : Inport
  fISENB : Inport  Port=2
  fISENC : Inport  Port=3
  Float to IQN2 : tiiqmathlib/Float to IQN  Q_value=18
      settings: SourceProductBaseCode=TIC2000
  Float to IQN3 : tiiqmathlib/Float to IQN  Q_value=18
      settings: SourceProductBaseCode=TIC2000
  Gain : Gain  Gain=2/3  OutDataTypeStr=fixdt(1,32,16)
  Gain1 : Gain  Gain=-1/3  OutDataTypeStr=fixdt(1,32,16)
  Gain2 : Gain  Gain=-1/3  OutDataTypeStr=fixdt(1,32,16)
  Gain3 : Gain  Gain=sqrt(3)/3  OutDataTypeStr=fixdt(1,32,16)
  Gain4 : Gain  Gain=-sqrt(3)/3  OutDataTypeStr=fixdt(1,32,16)
  Sum : Sum  Inputs=|+++  OutDataTypeStr=single
  Sum1 : Sum  Inputs=|++  AccumDataTypeStr=single  OutDataTypeStr=single
  fpIalfa : Outport
  fpIbeta : Outport  Port=2
  wires:
  Gain3/1 -> Sum1/1
  Gain4/1 -> Sum1/2
  Gain2/1 -> Sum/3
  Gain1/1 -> Sum/2
  fISENC/1 -> Gain4/1, Gain2/1
  Gain/1 -> Sum/1
  fISENB/1 -> Gain1/1, Gain3/1
  fISENA/1 -> Gain/1
  Float to IQN2/1 -> fpIalfa/1
  Float to IQN3/1 -> fpIbeta/1
  Sum1/1 -> Float to IQN3/1
  Sum/1 -> Float to IQN2/1

== system LICENTA_2024/Subsystem/transf park ==
  alpha : Inport
  beta : Inport  Port=2
  "teta " : Inport  Port=3
  IQN1 x IQN{,1..3} (4 alike) : tiiqmathlib/IQN1 x IQN2  Q=20
      settings: SourceProductName=Embedded Coder Support Package for Texas Instruments C2000 Processors  SourceProductBaseCode=TIC2000
  Sum3 : Sum  Inputs=|++
  Sum4 : Sum  Inputs=|-+
  cos : tiiqmathlib/Trig Fcn IQN  functionOption=_IQcos
      settings: SourceProductName=Embedded Coder Support Package for Texas Instruments C2000 Processors  SourceProductBaseCode=TIC2000
  sin : tiiqmathlib/Trig Fcn IQN  functionOption=_IQsin
      settings: SourceProductName=Embedded Coder Support Package for Texas Instruments C2000 Processors  SourceProductBaseCode=TIC2000
  d : Outport
  q : Outport  Port=2
  wires:
  Sum3/1 -> d/1
  Sum4/1 -> q/1
  "teta "/1 -> sin/1, cos/1
  IQN1 x IQN1/1 -> Sum3/1  "beta*sin(theta)"
  IQN1 x IQN2/1 -> Sum3/2  "alpha*cos(theta)"
  IQN1 x IQN3/1 -> Sum4/2  "beta*cos(theta)"
  IQN1 x IQN/1 -> Sum4/1  "alpha*sin(theta)"
  cos/1 -> IQN1 x IQN3/1, IQN1 x IQN2/2
  sin/1 -> IQN1 x IQN1/1, IQN1 x IQN/2
  alpha/1 -> IQN1 x IQN2/1, IQN1 x IQN/1
  beta/1 -> IQN1 x IQN1/2, IQN1 x IQN3/2

== system LICENTA_2024/Subsystem2/Park Inverse1 ==
  d : Inport
  q : Inport  Port=2
  teta : Inport  Port=3
  Data Type Conversion : DataTypeConversion  OutDataTypeStr=fixdt(1,32,20)
  Data Type Conversion1 : DataTypeConversion  OutDataTypeStr=fixdt(1,32,20)
  IQN1 x IQN{1..4} (4 alike) : tiiqmathlib/IQN1 x IQN2  Q=20
      settings: SourceProductName=Embedded Coder Support Package for Texas Instruments C2000 Processors  SourceProductBaseCode=TIC2000
  Sum1 : Sum  Inputs=|++  OutDataTypeStr=Inherit: Same as first input
  Sum2 : Sum  Inputs=|+-  OutDataTypeStr=Inherit: Same as first input
  cos IQN : tiiqmathlib/Trig Fcn IQN  functionOption=_IQcos
      settings: SourceProductName=Embedded Coder Support Package for Texas Instruments C2000 Processors  SourceProductBaseCode=TIC2000
  sin IQN : tiiqmathlib/Trig Fcn IQN  functionOption=_IQsin
      settings: SourceProductName=Embedded Coder Support Package for Texas Instruments C2000 Processors  SourceProductBaseCode=TIC2000
  alpha : Outport
  beta : Outport  Port=2
  wires:
  teta/1 -> cos IQN/1, sin IQN/1
  Sum2/1 -> alpha/1
  d/1 -> Data Type Conversion/1
  sin IQN/1 -> IQN1 x IQN4/2, IQN1 x IQN1/2
  cos IQN/1 -> IQN1 x IQN3/2, IQN1 x IQN2/2
  q/1 -> Data Type Conversion1/1
  Sum1/1 -> beta/1
  IQN1 x IQN2/1 -> Sum2/1
  IQN1 x IQN1/1 -> Sum2/2
  IQN1 x IQN3/1 -> Sum1/1
  IQN1 x IQN4/1 -> Sum1/2
  Data Type Conversion/1 -> IQN1 x IQN4/1, IQN1 x IQN2/1
  Data Type Conversion1/1 -> IQN1 x IQN3/1, IQN1 x IQN1/1

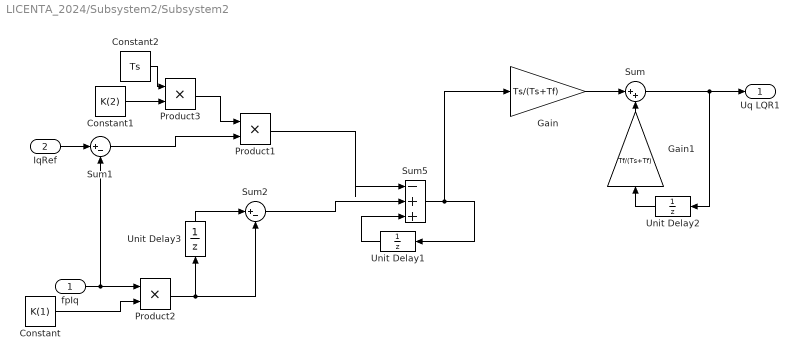
== system LICENTA_2024/Subsystem2/Subsystem2 ==
  fpIq : Inport
  IqRef : Inport  Port=2
  Constant : Constant  Value=K(1)
  Constant1 : Constant  Value=K(2)
  Constant2 : Constant  Value=Ts
  Gain : Gain  Gain=Ts/(Ts+Tf)
  Gain1 : Gain  Gain=Tf/(Ts+Tf)
  Product1 : Product
  Product2 : Product
  Product3 : Product
  Sum : Sum  Inputs=|++
  Sum1 : Sum  Inputs=|+-
  Sum2 : Sum  Inputs=|+-
  Sum5 : Sum  Inputs=|-++
  Unit Delay1 : UnitDelay  SampleTime=-1
  Unit Delay2 : UnitDelay  SampleTime=-1
  Unit Delay3 : UnitDelay  SampleTime=-1
  Uq LQR1 : Outport
  wires:
  Product1/1 -> Sum5/1
  fpIq/1 -> Product2/1, Sum1/2
  Product3/1 -> Product1/1
  Constant/1 -> Product2/2
  Constant2/1 -> Product3/1
  Unit Delay3/1 -> Sum2/1
  Product2/1 -> Unit Delay3/1, Sum2/2
  Unit Delay1/1 -> Sum5/3
  Constant1/1 -> Product3/2
  IqRef/1 -> Sum1/1
  Sum1/1 -> Product1/2
  Sum2/1 -> Sum5/2
  Gain1/1 -> Sum/2
  Gain/1 -> Sum/1
  Unit Delay2/1 -> Gain1/1
  Sum/1 -> Uq LQR1/1, Unit Delay2/1
  Sum5/1 -> Unit Delay1/1, Gain/1

== system LICENTA_2024/Subsystem2/Subsystem4 ==
  fpId : Inport
  IdRef : Inport  Port=2
  Constant : Constant  Value=K(1)
  Constant1 : Constant  Value=K(2)
  Constant2 : Constant  Value=Ts
  Gain : Gain  Gain=Ts/(Ts+Tf)
  Gain1 : Gain  Gain=Tf/(Ts+Tf)
  Product1 : Product
  Product2 : Product
  Product3 : Product
  Sum : Sum  Inputs=|++
  Sum1 : Sum  Inputs=|+-
  Sum2 : Sum  Inputs=|+-
  Sum5 : Sum  Inputs=|-++
  Unit Delay1 : UnitDelay  SampleTime=-1
  Unit Delay2 : UnitDelay  SampleTime=-1
  Unit Delay3 : UnitDelay  SampleTime=-1
  Ud LQR1 : Outport
  wires:
  Sum5/1 -> Unit Delay1/1, Gain/1
  Unit Delay1/1 -> Sum5/3
  Product2/1 -> Sum2/2, Unit Delay3/1
  Unit Delay3/1 -> Sum2/1
  Constant2/1 -> Product3/1
  Constant/1 -> Product2/2
  Product3/1 -> Product1/1
  fpId/1 -> Product2/1, Sum1/2
  Product1/1 -> Sum5/1
  Constant1/1 -> Product3/2
  IdRef/1 -> Sum1/1
  Sum1/1 -> Product1/2
  Sum2/1 -> Sum5/2
  Unit Delay2/1 -> Gain1/1
  Gain1/1 -> Sum/2
  Gain/1 -> Sum/1
  Sum/1 -> Ud LQR1/1, Unit Delay2/1

== system LICENTA_2024/Subsystem3/Subsystem5 ==
  "torque_Ref " : Inport
  Constant : Constant  Value=const_cuplu
  Product : Product  Inputs=*/
  Saturation : Saturate  UpperLimit=0.8  LowerLimit=-0.8
  IqRef : Outport
  wires:
  Product/1 -> Saturation/1
  "torque_Ref "/1 -> Product/1
  Constant/1 -> Product/2
  Saturation/1 -> IqRef/1

== system LICENTA_2024/Subsystem3/regulator curent iq ==
  KiPI : Inport
  KpPI : Inport  Port=2
  iqRef : Inport  Port=3
  fpiq : Inport  Port=4
  Constant : Constant  Value=T_pos  OutDataTypeStr=single  SampleTime=-1
  Gain : Gain  Commented=on  Gain=T_pos/(T_pos+Tf)
  Gain1 : Gain  Commented=on  Gain=Tf/(T_pos+Tf)
  Product{,1..3} (4 alike) : Product
  Sum : Sum  Commented=on  Inputs=|++
  Sum1 : Sum  Inputs=|+-
  Sum2 : Sum  Inputs=+-++
  Unit Delay1 : UnitDelay  Commented=on  SampleTime=-1
  Unit Delay2 : UnitDelay  SampleTime=-1
  Unit Delay3 : UnitDelay  SampleTime=-1
  Uq PI1 : Outport
  wires:
  Sum1/1 -> Product3/2, Product2/2, Unit Delay2/1
  fpiq/1 -> Sum1/2
  iqRef/1 -> Sum1/1
  KiPI/1 -> Product/1
  Constant/1 -> Product/2
  Sum2/1 -> Uq PI1/1, Unit Delay3/1
  Unit Delay3/1 -> Sum2/4
  Product2/1 -> Sum2/1
  KpPI/1 -> Product1/1, Product2/1
  Product1/1 -> Sum2/2
  Product3/1 -> Sum2/3
  Product/1 -> Product3/1
  Unit Delay2/1 -> Product1/2
  Unit Delay1/1 -> Gain1/1
  Gain/1 -> Sum/1
  Gain1/1 -> Sum/2
  Sum/1 -> Unit Delay1/1

== system LICENTA_2024/calc pozitiei si a vitezei/calc pozitie ==
  In1 : Inport
  Data Type Conversion : DataTypeConversion  OutDataTypeStr=int8
  MATLAB Function : MATLAB Function  TreatAsAtomicUnit=on
  citire senzori hall & calcul teta : Subsystem
  gradient : Subsystem
  teta : Outport  VectorParamsAs1DForOutWhenUnconnected=on
  int8dir : Outport  Port=2  VectorParamsAs1DForOutWhenUnconnected=on
  wires:
  Data Type Conversion/1 -> int8dir/1
  MATLAB Function/1(dir) -> Data Type Conversion/1
  gradient/1(gradient) -> MATLAB Function/1(u)
  citire senzori hall & calcul teta/1(teta) -> teta/1, gradient/1(teta)
  citire senzori hall & calcul teta/2("seq. change detected ") -> gradient/Trigger
  In1/1 -> citire senzori hall & calcul teta/1(In1)

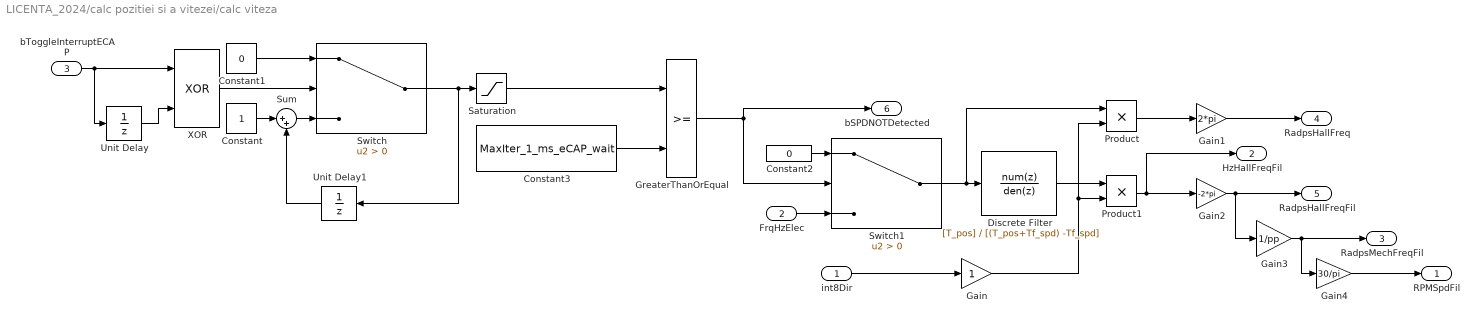
== system LICENTA_2024/calc pozitiei si a vitezei/calc viteza ==
  int8Dir : Inport
  FrqHzElec : Inport  Port=2
  bToggleInterruptECAP : Inport  Port=3
  Constant : Constant
  Constant1 : Constant  Value=0
  Constant2 : Constant  Value=0
  Constant3 : Constant  Value=MaxIter_1_ms_eCAP_wait
  Discrete Filter : DiscreteFilter  Numerator=[T_pos]  Denominator=[(T_pos+Tf_spd) -Tf_spd]
  Gain : Gain
  Gain1 : Gain  Gain=2*pi
  Gain2 : Gain  Gain=-2*pi
  Gain3 : Gain  Gain=1/pp
  Gain4 : Gain  Gain=30/pi
  GreaterThanOrEqual : RelationalOperator  OutDataTypeStr=boolean  RndMeth=Simplest
  Product : Product
  Product1 : Product
  Saturation : Saturate  UpperLimit=MaxIter_1_ms_eCAP_wait  LowerLimit=0
  Sum : Sum  Inputs=|++
  Switch : Switch  Criteria=u2 > Threshold
  Switch1 : Switch  Criteria=u2 > Threshold
  Unit Delay : UnitDelay  SampleTime=-1
  Unit Delay1 : UnitDelay  SampleTime=-1
  XOR : Logic  Operator=XOR  IconShape=distinctive  AllPortsSameDT=off  OutDataTypeStr=boolean
  RPMSpdFil : Outport  VectorParamsAs1DForOutWhenUnconnected=on
  HzHallFreqFil : Outport  Port=2  VectorParamsAs1DForOutWhenUnconnected=on
  RadpsMechFreqFil : Outport  Port=3  VectorParamsAs1DForOutWhenUnconnected=on
  RadpsHallFreq : Outport  Port=4  VectorParamsAs1DForOutWhenUnconnected=on
  RadpsHallFreqFil : Outport  Port=5  VectorParamsAs1DForOutWhenUnconnected=on
  bSPDNOTDetected : Outport  Port=6  VectorParamsAs1DForOutWhenUnconnected=on
  wires:
  Constant2/1 -> Switch1/1
  FrqHzElec/1 -> Switch1/3
  Sum/1 -> Switch/3
  Unit Delay/1 -> XOR/2
  Saturation/1 -> GreaterThanOrEqual/1
  bToggleInterruptECAP/1 -> XOR/1, Unit Delay/1
  Unit Delay1/1 -> Sum/2
  Switch/1 -> Unit Delay1/1, Saturation/1
  Constant/1 -> Sum/1
  Product1/1 -> Gain2/1, HzHallFreqFil/1
  XOR/1 -> Switch/2
  Product/1 -> Gain1/1
  Constant3/1 -> GreaterThanOrEqual/2
  Gain1/1 -> RadpsHallFreq/1
  Gain/1 -> Product1/2, Product/2
  Constant1/1 -> Switch/1
  Gain4/1 -> RPMSpdFil/1
  Gain2/1 -> Gain3/1, RadpsHallFreqFil/1
  GreaterThanOrEqual/1 -> Switch1/2, bSPDNOTDetected/1
  Gain3/1 -> Gain4/1, RadpsMechFreqFil/1
  Discrete Filter/1 -> Product1/1
  int8Dir/1 -> Gain/1
  Switch1/1 -> Product/1, Discrete Filter/1

== system LICENTA_2024/eCAP/If Action Subsystem ==
  HzHallFreqPrev : Inport
  Action Port : ActionPort  ActionType=then
  HzHallFreq : Outport  VectorParamsAs1DForOutWhenUnconnected=on
  wires:
  HzHallFreqPrev/1 -> HzHallFreq/1

== system LICENTA_2024/eCAP/If Action Subsystem1 ==
  Action Port : ActionPort  ActionType=elseif
  Constant : Constant  Value=0
  HzHallFreq : Outport  VectorParamsAs1DForOutWhenUnconnected=on
  wires:
  Constant/1 -> HzHallFreq/1

== system LICENTA_2024/eCAP/If Action Subsystem2 ==
  HallPeriod : Inport
  Action Port : ActionPort  ActionType=else
  Constant : Constant
  Multiply : Product  Inputs=*/
  HzHallFreq : Outport  VectorParamsAs1DForOutWhenUnconnected=on
  wires:
  HallPeriod/1 -> Multiply/2
  Constant/1 -> Multiply/1
  Multiply/1 -> HzHallFreq/1

== system LICENTA_2024/calc pozitiei si a vitezei/calc pozitie/citire senzori hall & calcul teta ==
  In1 : Inport
  Digital Input : c2837xDlib/Digital Input  GPIO_Number=GPIO24~GPIO31  GPIO_Bit0=off  GPIO_Bit1=off  GPIO_Bit2=on  GPIO_Bit3=off  GPIO_Bit4=off  GPIO_Bit5=off  GPIO_Bit6=off  GPIO_Bit7=off  sampleTime=-1  dataType=auto  GPIO_Bit0_Qualification=Sync to SYSCLKOUT  GPIO_Bit1_Qualification=Sync to SYSCLKOUT  GPIO_Bit2_Qualification=Sync to SYSCLKOUT  GPIO_Bit3_Qualification=Sync to SYSCLKOUT  GPIO_Bit4_Qualification=Sync to SYSCLKOUT  GPIO_Bit5_Qualification=Sync to SYSCLKOUT  GPIO_Bit6_Qualification=Sync to SYSCLKOUT  GPIO_Bit7_Qualification=Sync to SYSCLKOUT  Qualification_Period=-1
      settings: SourceProductBaseCode=TIC2000
  Digital Input1 : c2837xDlib/Digital Input  GPIO_Number=GPIO24~GPIO31  GPIO_Bit0=off  GPIO_Bit1=off  GPIO_Bit2=off  GPIO_Bit3=on  GPIO_Bit4=off  GPIO_Bit5=off  GPIO_Bit6=off  GPIO_Bit7=off  sampleTime=-1  dataType=auto  GPIO_Bit0_Qualification=Sync to SYSCLKOUT  GPIO_Bit1_Qualification=Sync to SYSCLKOUT  GPIO_Bit2_Qualification=Sync to SYSCLKOUT  GPIO_Bit3_Qualification=Sync to SYSCLKOUT  GPIO_Bit4_Qualification=Sync to SYSCLKOUT  GPIO_Bit5_Qualification=Sync to SYSCLKOUT  GPIO_Bit6_Qualification=Sync to SYSCLKOUT  GPIO_Bit7_Qualification=Sync to SYSCLKOUT  Qualification_Period=-1
      settings: SourceProductBaseCode=TIC2000
  Digital Input2 : c2837xDlib/Digital Input  GPIO_Number=GPIO24~GPIO31  GPIO_Bit0=off  GPIO_Bit1=on  GPIO_Bit2=off  GPIO_Bit3=off  GPIO_Bit4=off  GPIO_Bit5=off  GPIO_Bit6=off  GPIO_Bit7=off  sampleTime=-1  dataType=auto  GPIO_Bit0_Qualification=Sync to SYSCLKOUT  GPIO_Bit1_Qualification=Sync to SYSCLKOUT  GPIO_Bit2_Qualification=Sync to SYSCLKOUT  GPIO_Bit3_Qualification=Sync to SYSCLKOUT  GPIO_Bit4_Qualification=Sync to SYSCLKOUT  GPIO_Bit5_Qualification=Sync to SYSCLKOUT  GPIO_Bit6_Qualification=Sync to SYSCLKOUT  GPIO_Bit7_Qualification=Sync to SYSCLKOUT  Qualification_Period=-1
      settings: SourceProductBaseCode=TIC2000
  Optimizare : Subsystem
  transf clarke : Subsystem
  teta : Outport  VectorParamsAs1DForOutWhenUnconnected=on
  "seq. change detected " : Outport  Port=2
  wires:
  Digital Input2/1 -> transf clarke/1(HallA), Optimizare/1(HallA)
  Digital Input/1 -> transf clarke/2(HallB), Optimizare/2(HallB)
  Digital Input1/1 -> transf clarke/3(HallC), Optimizare/3(HallC)
  Optimizare/1("seq. change detected ") -> "seq. change detected "/1, transf clarke/Trigger
  transf clarke/1(teta) -> teta/1
  In1/1 -> transf clarke/4(teta_allighn)

== system LICENTA_2024/calc pozitiei si a vitezei/calc pozitie/gradient ==
  teta : Inport
  Trigger : TriggerPort  VariantControl=Variant  PortDimensions=1
  Sum : Sum  Inputs=+-
  Unit Delay : UnitDelay  SampleTime=-1
  gradient : Outport  VectorParamsAs1DForOutWhenUnconnected=on
  wires:
  Unit Delay/1 -> Sum/2
  Sum/1 -> gradient/1
  teta/1 -> Sum/1, Unit Delay/1

== system LICENTA_2024/calc pozitiei si a vitezei/calc pozitie/citire senzori hall & calcul teta/Optimizare ==
  HallA : Inport
  HallB : Inport  Port=2
  HallC : Inport  Port=3
  Unit Delay : UnitDelay  SampleTime=-1
  Unit Delay1 : UnitDelay  SampleTime=-1
  Unit Delay2 : UnitDelay  SampleTime=-1
  XOR : Logic  Operator=XOR  Inputs=6  AllPortsSameDT=off  OutDataTypeStr=boolean
  "seq. change detected " : Outport  VectorParamsAs1DForOutWhenUnconnected=on
  wires:
  XOR/1 -> "seq. change detected "/1
  Unit Delay1/1 -> XOR/6
  Unit Delay2/1 -> XOR/5
  HallC/1 -> XOR/3, Unit Delay1/1
  HallA/1 -> XOR/1, Unit Delay/1
  Unit Delay/1 -> XOR/4
  HallB/1 -> XOR/2, Unit Delay2/1

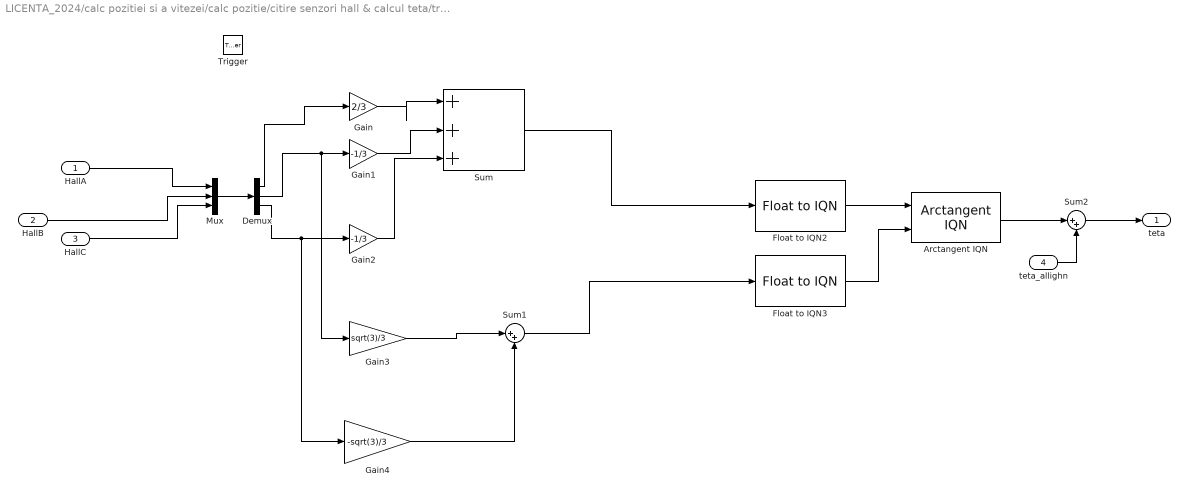
== system LICENTA_2024/calc pozitiei si a vitezei/calc pozitie/citire senzori hall & calcul teta/transf clarke ==
  HallA : Inport
  HallB : Inport  Port=2
  HallC : Inport  Port=3
  teta_allighn : Inport  Port=4
  Trigger : TriggerPort  VariantControl=(inherit)  PortDimensions=1
  Arctangent IQN : tiiqmathlib/Arctangent IQN  tanOption=atan2 (radians)
      settings: SourceProductBaseCode=TIC2000
  Demux : Demux  Outputs=3
  Float to IQN2 : tiiqmathlib/Float to IQN  Q_value=20
      settings: SourceProductBaseCode=TIC2000
  Float to IQN3 : tiiqmathlib/Float to IQN  Q_value=20
      settings: SourceProductBaseCode=TIC2000
  Gain : Gain  Gain=2/3
  Gain1 : Gain  Gain=-1/3
  Gain2 : Gain  Gain=-1/3
  Gain3 : Gain  Gain=sqrt(3)/3
  Gain4 : Gain  Gain=-sqrt(3)/3
  Mux : Mux  Inputs=3
  Sum : Sum  Inputs=|+++  OutDataTypeStr=single
  Sum1 : Sum  Inputs=|++  AccumDataTypeStr=single
  Sum2 : Sum  Inputs=|++
  teta : Outport  VectorParamsAs1DForOutWhenUnconnected=on
  wires:
  Mux/1 -> Demux/1
  HallC/1 -> Mux/3
  HallB/1 -> Mux/2
  HallA/1 -> Mux/1
  Gain3/1 -> Sum1/1
  Gain4/1 -> Sum1/2
  Gain2/1 -> Sum/3
  Gain1/1 -> Sum/2
  Demux/3 -> Gain2/1, Gain4/1
  Gain/1 -> Sum/1
  Demux/2 -> Gain1/1, Gain3/1
  Demux/1 -> Gain/1
  Float to IQN2/1 -> Arctangent IQN/1
  Float to IQN3/1 -> Arctangent IQN/2
  Sum1/1 -> Float to IQN3/1
  Sum/1 -> Float to IQN2/1
  Sum2/1 -> teta/1
  teta_allighn/1 -> Sum2/2
  Arctangent IQN/1 -> Sum2/1

== matlab function LICENTA_2024/calc pozitiei si a vitezei/calc pozitie/MATLAB Function ==
  data: u input; dir output
function dir = fcn(u)

persistent dir_prev;
if isempty(dir_prev)
    dir_prev=0;
end
if (u < -2 || u > 2)
    dir=dir_prev;
else
    if u > 0.5
        dir = 1;
    elseif u < -0.5
        dir = -1;
    else
        dir = 0;
    end
end
dir_prev=dir;
